simulink subsystem "Aviate"  (R2025b)
settings: Solver=VariableStepAuto  StartTime=0.0  StopTime=10.0  RelTol=1e-3
settings Model: Creator=invrt  LastModifiedBy=jordan

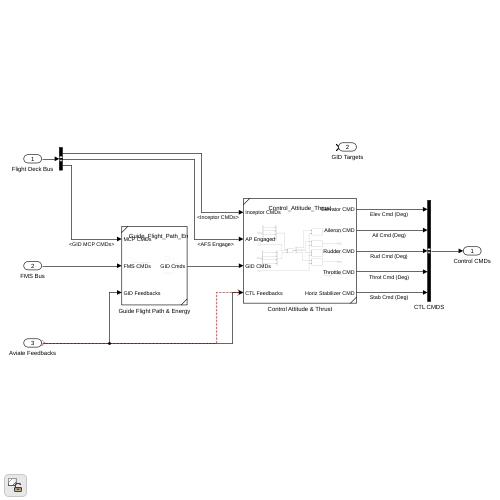
[thumbnail: Simulink's stored preview of the top-level diagram]
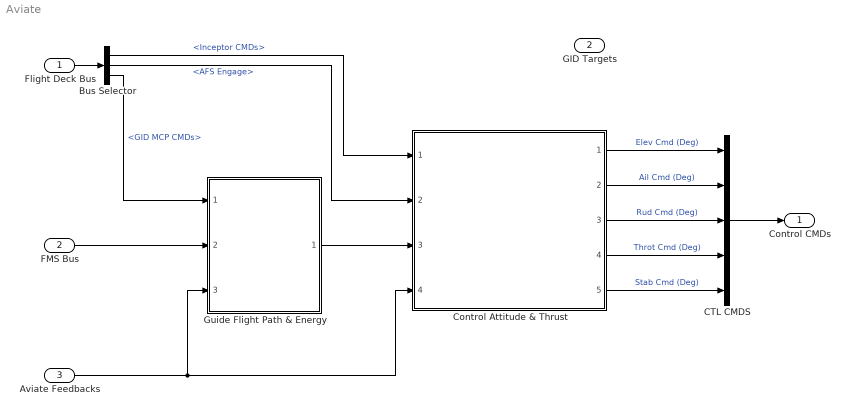
== system Aviate ==
  Flight Deck Bus : Inport
  FMS Bus : Inport  Port=2
  Aviate Feedbacks : Inport  Port=3
  Bus Selector : BusSelector  OutputSignals=Inceptor CMDs,GID MCP CMDs.AFS Engage,GID MCP CMDs
  CTL CMDS : BusCreator  Inputs=5
  Control Attitude & Thrust : Subsystem  ReferencedSubsystem=Control_Attitude_Thrust
  Guide Flight Path & Energy : Subsystem  ReferencedSubsystem=Guide_Flight_Path_Energy
  Control CMDs : Outport
  GID Targets : Outport  Port=2
  wires:
  CTL CMDS/1 -> Control CMDs/1
  Control Attitude & Thrust/1 -> CTL CMDS/1  "Elev Cmd (Deg)"
  Control Attitude & Thrust/2 -> CTL CMDS/2  "Ail Cmd (Deg)"
  Control Attitude & Thrust/3 -> CTL CMDS/3  "Rud Cmd (Deg)"
  Control Attitude & Thrust/4 -> CTL CMDS/4  "Throt Cmd (Deg)"
  FMS Bus/1 -> Guide Flight Path & Energy/2
  Flight Deck Bus/1 -> Bus Selector/1
  Bus Selector/1 -> Control Attitude & Thrust/1  "<Inceptor CMDs>"
  Bus Selector/3 -> Guide Flight Path & Energy/1  "<GID MCP CMDs>"
  Control Attitude & Thrust/5 -> CTL CMDS/5  "Stab Cmd (Deg)"
  Guide Flight Path & Energy/1 -> Control Attitude & Thrust/3
  Bus Selector/2 -> Control Attitude & Thrust/2  "<AFS Engage>"
  Aviate Feedbacks/1 -> Guide Flight Path & Energy/3, Control Attitude & Thrust/4
